simulink model "allin"  (R2024a)
settings: Solver=FixedStepAuto  StartTime=0.0  StopTime=60  FixedStep=1e-3  RelTol=1e-3
StopFcn:
  | % plot3(x,y,-z);
  | % xlabel('x');
  | % ylabel('y');
  | % zlabel('z');
  | % grid on;
undefined symbols (not defined in the file or in its folder): k_a_z, k_d_z, k_i_phi, k_i_psi, k_i_tt, k_i_x, k_i_y, k_i_z, k_p_phi, k_p_psi, k_p_tt, k_p_x, k_p_y, k_p_z
libraries: simulink x2
settings Model: Creator=luand  LastModifiedBy=luand
settings DataIOCC: ReturnWorkspaceOutputs=off
settings RTWCC: GPUComputeCapability=3.5

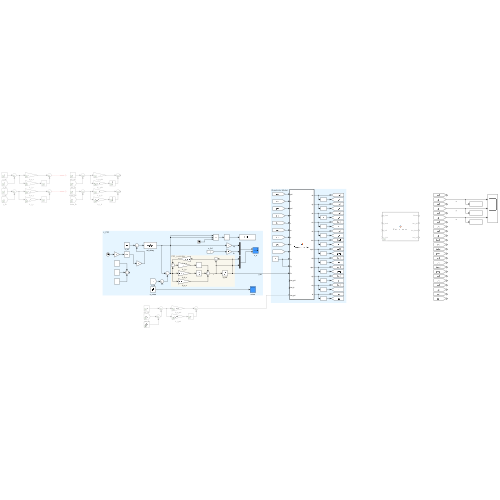
[thumbnail: Simulink's stored preview of the top-level diagram]
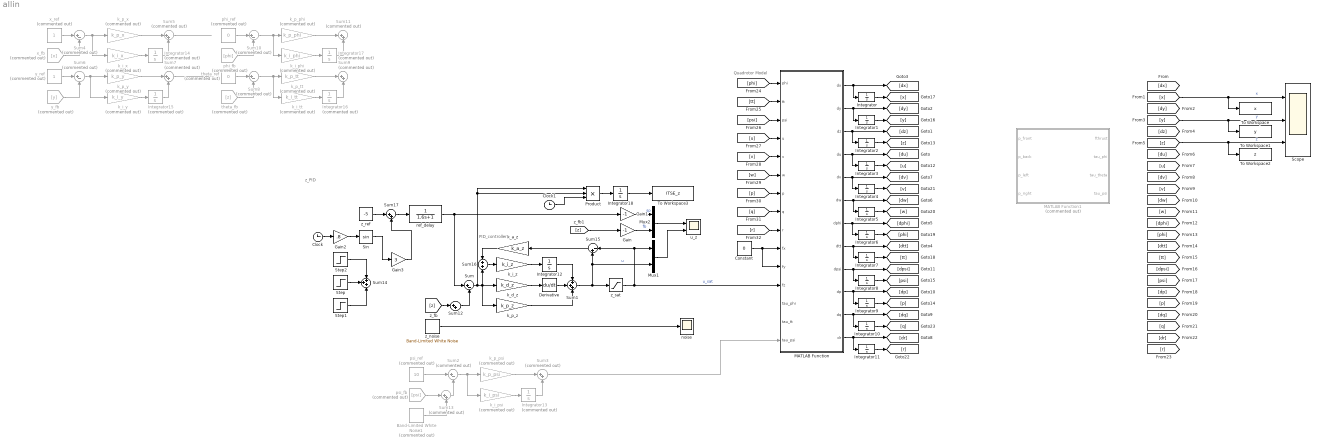
== system allin ==
  note: PID_controller
  note: z_PID
  note: Quadrotor Model
  Band-Limited White Noise1 : simulink/Sources/Band-Limited White Noise  Commented=on  Cov=[0.01]  Ts=0.1  seed=[23341]
  Clock : Clock
  Clock1 : Clock
  Constant : Constant  Value=0
  Derivative : Derivative
  Gain : Gain  Gain=-1
  Gain1 : Gain  Gain=-1
  Gain2 : Gain  Gain=.8
  Gain3 : Gain  Gain=3
  Integrator{,1,3..11,18} (12 alike) : Integrator
  Integrator12 : Integrator  UpperSaturationLimit=10000  LowerSaturationLimit=-10000
  Integrator{13..17} (5 alike) : Integrator  Commented=on
  Integrator2 : Integrator  LimitOutput=on  UpperSaturationLimit=0  LowerSaturationLimit=-1000
  MATLAB Function : MATLAB Function  TreatAsAtomicUnit=on
  MATLAB Function1 : MATLAB Function  Commented=on  TreatAsAtomicUnit=on
  Mux1 : Mux  Inputs=2
  Mux2 : Mux  Inputs=2
  Product : Product  Inputs=3
  Scope : Scope  NumInputPorts=3
  Sin : Trigonometry
  Step : Step  Time=25  After=-20  SampleTime=0
  Step1 : Step  Time=40  After=15  SampleTime=0
  Step2 : Step  Time=10  After=-5  SampleTime=0
  Sum : Sum  Inputs=|+-
  Sum1 : Sum  Inputs=+++
  Sum{2,4,6,8,10} (5 alike) : Sum  Commented=on  Inputs=|+-
  Sum{3,5,7,9,11,13} (6 alike) : Sum  Commented=on  Inputs=|++
  Sum12 : Sum  Inputs=|++
  Sum14 : Sum  Inputs=+++
  Sum15 : Sum  Inputs=|-+
  Sum16 : Sum  Inputs=+|+
  Sum17 : Sum  Inputs=|++
  To Workspace : ToWorkspace  VariableName=x  SampleTime=-1
      settings: Save2DSignal=2-D array (concatenate along first dimension)
  To Workspace1 : ToWorkspace  VariableName=y  SampleTime=-1
      settings: Save2DSignal=2-D array (concatenate along first dimension)
  To Workspace2 : ToWorkspace  VariableName=z  SampleTime=-1
      settings: Save2DSignal=2-D array (concatenate along first dimension)
  To Workspace3 : ToWorkspace  VariableName=ITSE_z  SampleTime=-1
  k_a_z : Gain  Gain=k_a_z
  k_d_z : Gain  Gain=k_d_z
  k_i_phi : Gain  Commented=on  Gain=k_i_phi
  k_i_psi : Gain  Commented=on  Gain=k_i_psi
  k_i_tt : Gain  Commented=on  Gain=k_i_tt
  k_i_x : Gain  Commented=on  Gain=k_i_x
  k_i_y : Gain  Commented=on  Gain=k_i_y
  k_i_z : Gain  Gain=k_i_z
  k_p_phi : Gain  Commented=on  Gain=k_p_phi
  k_p_psi : Gain  Commented=on  Gain=k_p_psi
  k_p_tt : Gain  Commented=on  Gain=k_p_tt
  k_p_x : Gain  Commented=on  Gain=k_p_x
  k_p_y : Gain  Commented=on  Gain=k_p_y
  k_p_z : Gain  Gain=k_p_z
  noise : Scope
  phi_fb : From  Commented=on  GotoTag=phi
  phi_ref : Constant  Commented=on  Value=0
  psi_fb : From  Commented=on  GotoTag=psi
  psi_ref : Constant  Commented=on  Value=10
  ref_delay : TransferFcn  Denominator=[1.6 1]
  theta_fb : From  Commented=on  GotoTag=z
  theta_ref : Constant  Commented=on  Value=0
  u_z : Scope  NumInputPorts=2
  x_fb : From  Commented=on  GotoTag=x
  x_ref : Constant  Commented=on
  y_fb : From  Commented=on  GotoTag=y
  y_ref : Constant  Commented=on
  z_noise : simulink/Sources/Band-Limited White Noise  Cov=[0.01]  Ts=0.1  seed=[23341]
  z_ref : Constant  Value=-5
  z_sat : Saturate  UpperLimit=60  LowerLimit=0
  wires:
  MATLAB Function/12(dr) -> Integrator11/1, [dr]
  MATLAB Function/11(dq) -> Integrator10/1, [dq]
  MATLAB Function/10(dp) -> Integrator9/1, [dp]
  MATLAB Function/9(dpsi) -> Integrator8/1, [dpsi]
  MATLAB Function/8(dtt) -> Integrator7/1, [dtt]
  MATLAB Function/7(dphi) -> Integrator6/1, [dphi]
  MATLAB Function/6(dw) -> Integrator5/1, [dw]
  MATLAB Function/5(dv) -> Integrator4/1, [dv]
  MATLAB Function/4(du) -> Integrator3/1, [du]
  MATLAB Function/3(dz) -> Integrator2/1, [dz]
  MATLAB Function/2(dy) -> Integrator1/1, [dy]
  MATLAB Function/1(dx) -> Integrator/1, [dx]
  Integrator/1 -> [x]
  Integrator1/1 -> [y]
  Integrator3/1 -> [u]
  Integrator2/1 -> [z]
  Integrator4/1 -> [v]
  Integrator5/1 -> [w]
  Integrator6/1 -> [phi]
  Integrator7/1 -> [tt]
  Integrator8/1 -> [psi]
  Integrator9/1 -> [p]
  Integrator10/1 -> [q]
  Integrator11/1 -> [r]
  [phi] -> MATLAB Function/1(phi)
  [tt] -> MATLAB Function/2(tt)
  [psi] -> MATLAB Function/3(psi)
  [u] -> MATLAB Function/4(u)
  [v] -> MATLAB Function/5(v)
  [w] -> MATLAB Function/6(w)
  [p] -> MATLAB Function/7(p)
  [x] -> Scope/1, To Workspace/1  "x"
  [y] -> Scope/2, To Workspace1/1  "y"
  [z] -> Scope/3, To Workspace2/1  "z"
  [q] -> MATLAB Function/8(q)
  [r] -> MATLAB Function/9(r)
  k_i_z/1 -> Integrator12/1
  Integrator13/1 -> Sum3/2
  k_p_psi/1 -> Sum3/1
  k_i_psi/1 -> Integrator13/1
  Sum2/1 -> k_p_psi/1, k_i_psi/1
  Integrator14/1 -> Sum5/2
  k_p_x/1 -> Sum5/1
  x_fb/1 -> Sum4/2
  x_ref/1 -> Sum4/1
  k_i_x/1 -> Integrator14/1
  Sum5/1 -> ?
  Sum4/1 -> k_p_x/1, k_i_x/1
  Integrator15/1 -> Sum7/2
  k_p_y/1 -> Sum7/1
  y_fb/1 -> Sum6/2
  y_ref/1 -> Sum6/1
  k_i_y/1 -> Integrator15/1
  Sum7/1 -> ?
  Sum6/1 -> k_p_y/1, k_i_y/1
  Sum10/1 -> k_p_phi/1, k_i_phi/1
  k_i_phi/1 -> Integrator17/1
  phi_ref/1 -> Sum10/1
  phi_fb/1 -> Sum10/2
  k_p_phi/1 -> Sum11/1
  Integrator17/1 -> Sum11/2
  Integrator16/1 -> Sum9/2
  k_p_tt/1 -> Sum9/1
  theta_fb/1 -> Sum8/2
  Sum8/1 -> k_p_tt/1, k_i_tt/1
  theta_ref/1 -> Sum8/1
  k_i_tt/1 -> Integrator16/1
  Constant/1 -> MATLAB Function/11(fy), MATLAB Function/10(fx)
  [z] -> Sum12/1
  Sum12/1 -> Sum/2
  psi_fb/1 -> Sum13/1
  Sum13/1 -> Sum2/2
  Band-Limited White Noise1/1 -> Sum13/2
  Clock/1 -> Gain2/1
  Gain2/1 -> Sin/1
  Step/1 -> Sum14/2
  Step2/1 -> Sum14/1
  Step1/1 -> Sum14/3
  Sum3/1 -> MATLAB Function/15(tau_psi)
  Sum/1 -> Product/1, Product/2, k_d_z/1, k_p_z/1, Sum16/2
  Sum1/1 -> Sum15/2, Mux1/2, z_sat/1  "u"
  z_sat/1 -> Sum15/1, Mux1/1, MATLAB Function/12(fz)  "u_sat"
  Sum16/1 -> k_i_z/1
  Sum15/1 -> k_a_z/1
  k_p_z/1 -> Sum1/3
  Integrator12/1 -> Sum1/1
  k_d_z/1 -> Derivative/1
  psi_ref/1 -> Sum2/1
  Product/1 -> Integrator18/1
  Clock1/1 -> Product/3
  Integrator18/1 -> To Workspace3/1
  k_a_z/1 -> Sum16/1
  Gain1/1 -> Mux2/1  "sp"
  Gain/1 -> Mux2/2  "fb"
  Mux2/1 -> u_z/1
  Mux1/1 -> u_z/2
  Derivative/1 -> Sum1/2
  ref_delay/1 -> Sum/1, Gain1/1
  Sum17/1 -> ref_delay/1
  z_noise/1 -> noise/1
  [z] -> Gain/1
  Sin/1 -> Gain3/1
  Gain3/1 -> Sum17/2
  z_ref/1 -> Sum17/1

== matlab function allin/MATLAB Function1 ==
  data: fthrust output; tau_phi output; tau_theta output; tau_psi output; p_front input; p_back input; p_left input; p_right input
function [fthrust, tau_phi, tau_theta, tau_psi] = Motor_dynamics(p_front, p_back, p_left, p_right)

fthrust = k_thrust*(p_front+p_back+p_left+p_right);
tau_phi = l*k_thrust*(-p_right+p_left);
tau_theta = l*k_thrust*(p_front+p_back);
tau_psi = k_momen*(-p_front-p_back+p_left+p_right);

== matlab function allin/MATLAB Function ==
  data: phi input; tt input; psi input; u input; dx output; v input; w input; p input; q input; r input; fx input; fy input; fz input; tau_phi input; tau_tt input; tau_psi input; dy output; dz output; du output; dv output; dw output; dphi output; dtt output; dpsi output; dp output; dq output; dr output
function [dx,dy,dz,du,dv,dw,dphi,dtt,dpsi,dp,dq,dr]=Dynamics_plustype(phi,tt,psi,u,v,w,p,q,r,fx,fy,fz,tau_phi,tau_tt,tau_psi)

% Eqs. 16-19

M = .75;
m = .05;
g = 9.81;
R = .03;
l = .22;

Jx = .4*M*R*R+2*l*l*m;
Jy = .4*M*R*R+2*l*l*m;
Jz = .4*M*R*R+4*l*l*m;

dx = cos(tt)*cos(psi)*u+(sin(phi)*sin(tt)*cos(psi)-cos(phi)*sin(psi))*v+(cos(phi)*sin(tt)*cos(psi)+sin(phi)*sin(psi))*w;
dy = cos(tt)*sin(psi)*u+(sin(phi)*sin(tt)*sin(psi)+cos(phi)*cos(psi))*v+(cos(phi)*sin(tt)*sin(psi)-sin(phi)*cos(psi))*w;
dz = -(sin(tt)*u-sin(phi)*cos(tt)*v-cos(phi)*cos(tt)*w);

du = (r*v-q*w)-g*sin(tt);
dv = (p*w-r*u)+g*cos(tt)*sin(phi);
dw = (q*u-p*v)+g*cos(tt)*cos(phi)-fz/(M+4*m);

dphi = p+sin(phi)*tan(phi)*q+cos(phi)*tan(tt)*r;
dtt  = cos(phi)*q-sin(phi)*r;
dpsi = sin(phi)*q/cos(tt)+cos(phi)*r/cos(tt);

dp = ((Jy-Jz)*q*r+tau_phi)/Jx;
dq = ((Jz-Jx)*p*r+tau_tt)/Jy;
dr = ((Jx-Jy)*q*p+tau_psi)/Jz;
